simulink model "DC_control"  (R2016a)
settings: Solver=ode45  SolverMode=SingleTasking  StartTime=0.0  StopTime=10.0  MaxStep=1e-3  RelTol=1e-3
values from neighbouring files (symbols this model uses):
  cam_angle = 140    [Model.m]
  D_regulator = 0.05    [Model.m]
  fs = 60    [Model.m]
  I_D_regulator = 3e-3    (= 0.003)    [Model.m]
  I_regulator = 0.1    [Model.m]
  imp_0 = 6000    [Model.m]
  imp_90 = 2000    [Model.m]
  K = 1/4.5/T    (= 4.44444444444)    [Model.m]
  K_regulator = 0.4    [Model.m]
  W_SIZE = 1280    [Model.m]
libraries: simulink x3, cstblocks x1
settings Model: Creator=plcrcmatlab4  LastModifiedBy=Marcin
settings SolverCC: EnableConcurrentExecution=on
settings DataIOCC: LimitDataPoints=on  SaveFormat=StructureWithTime
settings OptimizationCC: DefaultParameterBehavior=Inlined  UseDivisionForNetSlopeComputation=on  UseFloatMulNetSlope=on  InlineInvariantSignals=on  EfficientFloat2IntCast=on  OptimizeModelRefInitCode=on  LifeSpan=1
settings DebuggingCC: UnderspecifiedInitializationDetection=Classic  MergeDetectMultiDrivingBlocksExec=none  SolverPrmCheckMsg=warning  UnconnectedInputMsg=error  UnconnectedOutputMsg=error  UnconnectedLineMsg=error
settings HardwareCC: ProdBitPerPointer=32  ProdLargestAtomicInteger=Long  ProdLargestAtomicFloat=Double  ProdWordSize=32  ProdHWDeviceType=ARM Compatible->ARM Cortex
settings ModelReferenceCC: PropagateSignalLabelsOutOfModel=off
settings RTWCC: SystemTargetFile=ert.tlc  GenCodeOnly=on  TemplateMakefile=ert_default_tmf  GenerateReport=on  IncludeHyperlinkInReport=on  LaunchReport=on  GenerateTraceInfo=on  GenerateTraceReport=on  GenerateTraceReportSl=on  GenerateTraceReportSf=on  GenerateTraceReportEml=on  RTWCompilerOptimization=on
settings CodeAppCC: ForceParamTrailComments=on  IgnoreCustomStorageClasses=off  OperatorAnnotations=on  SimulinkDataObjDesc=on  SFDataObjDesc=on  MATLABFcnDesc=on  InsertBlockDesc=on  MATLABSourceComments=on
settings ERTTargetCC: GenerateSampleERTMain=on  InlinedParameterPlacement=NonHierarchical  ERTCustomFileTemplate=example_file_process.tlc
settings ConfigComp: CovModelRefEnable=Off

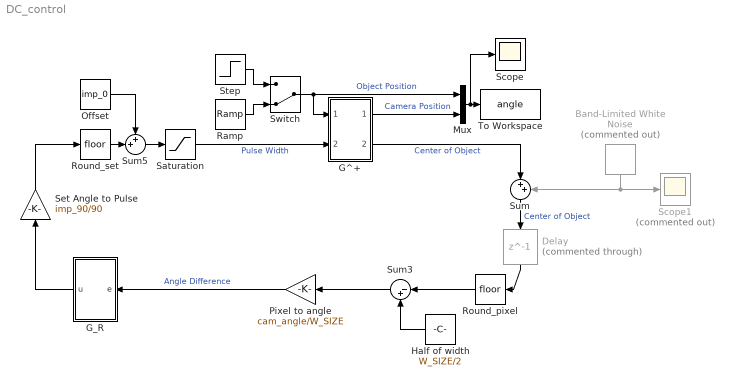
== system DC_control ==
  Band-Limited White Noise : simulink/Sources/Band-Limited White Noise  Commented=on  Cov=5  Ts=1/60  seed=[23341]
  Delay : Delay  Commented=through  DelayLength=1
  G^+ : Subsystem
      mask Display: disp('G^+(z)','texmode','on');
  G_R : Subsystem
      mask Display: disp('G_R(z)','interpreter','tex');
  Half of width : Constant  Value=W_SIZE/2
  Mux : Mux  Inputs=2
  Offset : Constant  Value=imp_0
  Pixel to angle : Gain  Gain=cam_angle/W_SIZE
  Ramp : simulink/Sources/Ramp  slope=30  start=0  X0=0
  Round_pixel : Rounding
  "Round_set " : Rounding
  Saturation : Saturate  UpperLimit=8000  LowerLimit=4000
  Scope : Scope
  Scope1 : Scope  Commented=on
  Set Angle to Pulse : Gain  Gain=imp_90/90  RndMeth=Nearest
  Step : Step  Time=0  After=30  SampleTime=0
  Sum : Sum  Inputs=|++
  Sum3 : Sum  Inputs=|-+
  Sum5 : Sum  Inputs=++|
  Switch : ManualSwitch  CurrentSetting=0
  To Workspace : ToWorkspace  VariableName=angle  SaveFormat=Timeseries  SampleTime=-1
  wires:
  Switch/1 -> G^+/1(In1), Mux/1  "Object Position"
  Half of width/1 -> Sum3/2
  Sum3/1 -> Pixel to angle/1
  Sum/1 -> Delay/1  "Center of Object"
  Mux/1 -> Scope/1, To Workspace/1
  Offset/1 -> Sum5/1
  Round_pixel/1 -> Sum3/1
  "Round_set "/1 -> Sum5/2
  Set Angle to Pulse/1 -> "Round_set "/1
  Pixel to angle/1 -> G_R/1(e)  "Angle Difference"
  G_R/1(u) -> Set Angle to Pulse/1
  Sum5/1 -> Saturation/1
  Saturation/1 -> G^+/2(In2)  "Pulse Width"
  G^+/1(Out1) -> Mux/2  "Camera Position"
  Ramp/1 -> Switch/2
  Step/1 -> Switch/1
  G^+/2(Out2) -> Sum/1  "Center of Object"
  Band-Limited White Noise/1 -> Scope1/1, Sum/2
  Delay/1 -> Round_pixel/1

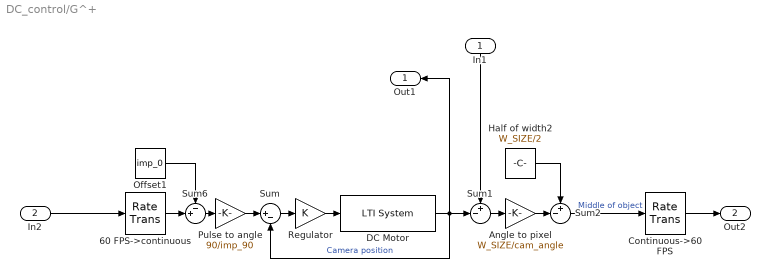
== system DC_control/G^+ ==
  In1 : Inport
  In2 : Inport  Port=2
  60 FPS->continuous : RateTransition  Deterministic=off  X0=6000
  Angle to pixel : Gain  Gain=W_SIZE/cam_angle
  Continuous->60 FPS : RateTransition  X0=640  OutPortSampleTime=1/60
  DC Motor : cstblocks/LTI System  sys=dc  IC=[]
  Half of width2 : Constant  Value=W_SIZE/2
  Offset1 : Constant  Value=imp_0
  Pulse to angle : Gain  Gain=90/imp_90
  Regulator : Gain  Gain=K
  Sum : Sum  Inputs=|+-
  Sum1 : Sum  Inputs=+-|
  Sum2 : Sum  Inputs=+-|
  Sum6 : Sum  Inputs=-+|
  Out1 : Outport
  Out2 : Outport  Port=2
  wires:
  In1/1 -> Sum1/1
  Offset1/1 -> Sum6/1
  DC Motor/1 -> Out1/1, Sum1/2, Sum/2  "Camera position"
  Pulse to angle/1 -> Sum/1
  Sum2/1 -> Continuous->60 FPS/1  "Middle of object"
  Sum6/1 -> Pulse to angle/1
  Half of width2/1 -> Sum2/1
  Angle to pixel/1 -> Sum2/2
  Regulator/1 -> DC Motor/1
  In2/1 -> 60 FPS->continuous/1
  Sum/1 -> Regulator/1
  60 FPS->continuous/1 -> Sum6/2
  Sum1/1 -> Angle to pixel/1
  Continuous->60 FPS/1 -> Out2/1

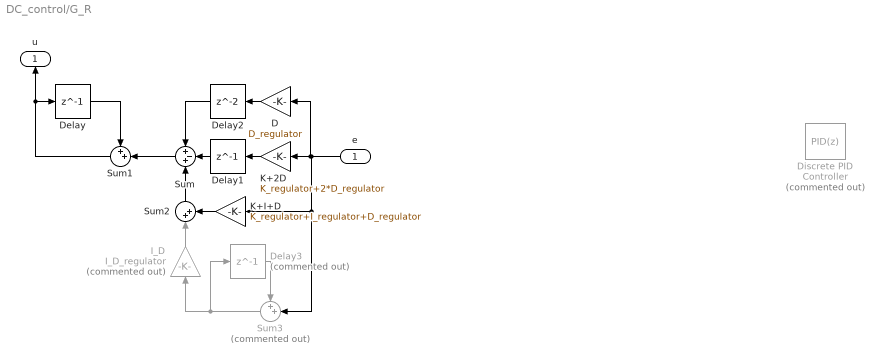
== system DC_control/G_R ==
  e : Inport
  D : Gain  Gain=D_regulator
  Delay : Delay  DelayLength=1
  Delay1 : Delay  DelayLength=1
  Delay2 : Delay
  Delay3 : Delay  Commented=on  DelayLength=1
  Discrete PID Controller : simulink/Continuous/PID Controller  Commented=on  Controller=PID  TimeDomain=Discrete-time  SampleTime=-1  IntegratorMethod=Backward Euler  FilterMethod=Forward Euler  Form=Parallel  UseFilter=off  ControllerParametersSource=internal  P=K_regulator  I=I_regulator*fs  D=D_regulator/fs  N=100  InitialConditionSource=internal  InitialConditionForIntegrator=0  InitialConditionForFilter=0  ExternalReset=none  LimitOutput=off  UpperSaturationLimit=inf  LowerSaturationLimit=-inf  LinearizeAsGain=off  AntiWindupMode=none  Kb=1  TrackingMode=off  Kt=1  PParamMin=[]  PParamMax=[]  IParamMin=[]  IParamMax=[]  DParamMin=[]  DParamMax=[]  NParamMin=[]  NParamMax=[]  KbParamMin=[]  KbParamMax=[]  KtParamMin=[]  KtParamMax=[]  POutMin=[]  POutMax=[]  IOutMin=[]  IOutMax=[]  DOutMin=[]  DOutMax=[]  NOutMin=[]  NOutMax=[]  KbOutMin=[]  KbOutMax=[]  KtOutMin=[]  KtOutMax=[]  IntegratorOutMin=[]  IntegratorOutMax=[]  FilterOutMin=[]  FilterOutMax=[]  SumOutMin=[]  SumOutMax=[]  SumI1OutMin=[]  SumI1OutMax=[]  SumI2OutMin=[]  SumI2OutMax=[]  SumI3OutMin=[]  SumI3OutMax=[]  SumDOutMin=[]  SumDOutMax=[]  SaturationOutMin=[]  SaturationOutMax=[]  IntegratorContinuousStateAttributes=''  IntegratorStateMustResolveToSignalObject=off  IntegratorRTWStateStorageClass=Auto  FilterContinuousStateAttributes=''  FilterStateMustResolveToSignalObject=off  FilterRTWStateStorageClass=Auto  DifferentiatorICPrevScaledInput=0  DifferentiatorOutMin=[]  DifferentiatorOutMax=[]
  I_D : Gain  Commented=on  Gain=I_D_regulator
  K+2D : Gain  Gain=K_regulator+2*D_regulator
  K+I+D : Gain  Gain=K_regulator+I_regulator+D_regulator
  Sum : Sum  Inputs=+-+
  Sum1 : Sum  Inputs=++|
  Sum2 : Sum  Inputs=|++
  Sum3 : Sum  Commented=on  Inputs=++|
  u : Outport
  wires:
  Delay/1 -> Sum1/1
  Sum1/1 -> u/1, Delay/1
  Delay1/1 -> Sum/2
  K+2D/1 -> Delay1/1
  Sum/1 -> Sum1/2
  D/1 -> Delay2/1
  Delay2/1 -> Sum/1
  e/1 -> Sum3/2, K+I+D/1, D/1, K+2D/1
  K+I+D/1 -> Sum2/2
  Sum2/1 -> Sum/3
  I_D/1 -> Sum2/1
  Sum3/1 -> Delay3/1, I_D/1
  Delay3/1 -> Sum3/1
